simulink model "Thesis_MMC_WF_Modify"  (R2023a)
settings: Solver=VariableStepAuto  StartTime=0.0  StopTime=16  RelTol=1e-3
InitFcn:
  | % TS %
  | Ts_Control=4e-05;
  | Ts_Power=2e-05;
  | %% Main Circuit %%
  | % AC Line %
  | Vnom_Sec=333000;
  | Vnom_Pri=400000;
  | Pnom=1.0e+09;
  | Fnom=60;
  | Psc=2.0e+10;
  | P_Ld1=2/3*1e+09;
  | R_Startup=400;
  | Rxfo=0.003;
  | Lxfo=0.12;
  | P_Ld2=500e+03;
  | % MMC Parameter %
  | Larm_pu=0.15;
  | Rarm_pu=Larm_pu/100;
  | Zbase= Vnom_Sec^2/Pnom;
  | Larm=Larm_pu*(Zbase/(2*pi*Fnom));
  | Rarm=Rarm_pu*Zbase;
  | C_PM=1.758e-3;
  | w=2*pi*Fnom;
  | wc2=(2*w)^2;
  | Cfilter=1/(Larm*wc2);
  | Rfilter=1/(Cfilter*w)*30;
  | Topen_Filter=1e6;
  | K_V_dc=600000;
  | n=36;
  | Rg=100;
  | Cg=5e-08;
  | % HVDC Parameter %
  | R_cable=0.5;
  | L_cable=0.015;
  | %% Controller Parameter %%
  | % PLL %
  | Fn_filter=1000;
  | Zeta_filter=1;
  | % Active Power Regulator %
  | Kp_Preg=1/6;
  | Ki_Preg=1;
  | Limits_Preg=[0.8 1.2];
  | set_param('Thesis_MMC_WF_Modify/Controller/Active Power Regulator/Sum1','SampleTime','Ts_Control')
  | set_param('Thesis_MMC_WF_Modify/Controller/Active Power Regulator/Saturation','SampleTime','Ts_Control')
  | % Reactive Power Regulator %
  | Kp_Qreg=1/6;
  | Ki_Qreg=1;
  | Limits_Qreg=[-0.25 0.25];
  | set_param('Thesis_MMC_WF_Modify/Controller/Reactive Power Regulartor/Sum1','SampleTime','Ts_Control')
  | % Discrete Mean %
  | K1=3.2312e-30;
  | K2=-1.1369e-16;
  | Delay=0.02;
  | Vint=0;
  | Delay1=0.02004;
  | % DC Voltage Regulator %
  | Kp_VDCreg=4;
  | Ki_VDCreg=100;
  | Limits_VDCreg=[-2 2];
  | set_param('Thesis_MMC_WF_Modify/Controller/DC Voltage Regulator/Sum1','SampleTime','Ts_Control')
  | ... (+46 lines)
undefined symbols (not defined in the file): D1, Delta, Delta1, DiscIntNeverNeededParam, Lagging, Vnom_dc
libraries: spsSeriesRLCBranchLib x54, spsIGBTLib x24, spsBreakerLib x13, spsVoltageMeasurementLib x11, spsThreePhaseBreakerLib x11, spsThreePhaseVIMeasurementLib x9, spsIdealSwitchLib x8, simulink x7, spsDiscreteVariableTimeDelayLib x7, spsCurrentMeasurementLib x6, spsGroundLib x6, spsSecondOrderFilterLib x6
(part 3 of 3)

== system Thesis_MMC_WF_Modify/Controller/Current Regular/PI Regulator2 ==
  Error : Inport
  Compare To Zero : simulink/Logic and Bit Operations/Compare To Zero  relop=>  OutDataTypeStr=uint8  ZeroCross=off
  Compare To Zero1 : simulink/Logic and Bit Operations/Compare To Zero  relop=<  OutDataTypeStr=uint8  ZeroCross=off
  Constant : Constant  Value=UpperLimit
  Constant1 : Constant  Value=0
  Constant2 : Constant  Value=LowerLimit
  Discrete-Time Integrator : DiscreteIntegrator  IntegratorMethod=Integration: Trapezoidal  SampleTime=Ts_Control  LimitOutput=on  UpperSaturationLimit=UpperLimit  LowerSaturationLimit=LowerLimit  ShowStatePort=on  ICPrevOutput=DiscIntNeverNeededParam  ICPrevScaledInput=DiscIntNeverNeededParam
  Gain1 : Gain  SampleTime=Ts_Control
  Gain2 : Gain  Gain=Ki  SampleTime=Ts_Control
  Logical Operator : Logic  AllPortsSameDT=off  OutDataTypeStr=boolean
  Logical Operator1 : Logic  Operator=OR  AllPortsSameDT=off  OutDataTypeStr=boolean
  Logical Operator2 : Logic  AllPortsSameDT=off  OutDataTypeStr=boolean
  Relational Operator : RelationalOperator  Operator=<=  OutDataTypeStr=boolean  RndMeth=Simplest  InputSameDT=off
  Relational Operator1 : RelationalOperator  OutDataTypeStr=boolean  RndMeth=Simplest  InputSameDT=off
  Saturation : Saturate  UpperLimit=UpperLimit  LowerLimit=LowerLimit  SampleTime=Ts_Control
  Sum1 : Sum  SampleTime=Ts_Control
  Sum2 : Sum  SampleTime=Ts_Control
  Switch : Switch  Criteria=u2 > Threshold  SaturateOnIntegerOverflow=off  InputSameDT=off
  Zero-Order Hold : ZeroOrderHold  SampleTime=Ts_Control
  Out : Outport
  wires:
  Constant1/1 -> Switch/1
  Gain2/1 -> Switch/3
  Gain1/1 -> Zero-Order Hold/1
  Error/1 -> Compare To Zero1/1, Compare To Zero/1, Gain2/1, Gain1/1
  Switch/1 -> Discrete-Time Integrator/1
  Zero-Order Hold/1 -> Sum1/1, Sum2/2
  Discrete-Time Integrator/1 -> Sum1/2
  Sum1/1 -> Saturation/1
  Saturation/1 -> Out/1
  Sum2/1 -> Relational Operator/1, Relational Operator1/1
  Discrete-Time Integrator/State -> Sum2/1
  Constant/1 -> Relational Operator1/2
  Constant2/1 -> Relational Operator/2
  Logical Operator1/1 -> Switch/2
  Compare To Zero/1 -> Logical Operator/2
  Compare To Zero1/1 -> Logical Operator2/2
  Relational Operator1/1 -> Logical Operator/1
  Relational Operator/1 -> Logical Operator2/1
  Logical Operator2/1 -> Logical Operator1/1
  Logical Operator/1 -> Logical Operator1/2

== system Thesis_MMC_WF_Modify/Controller/PLL,Measurement and Transformation/Discrete Mean ==
  In : Inport
  Constant : Constant  Value=Delay
  Constant1 : Constant  Value=Fnom  SampleTime=Ts_Control
  Constant2 : Constant  Value=Vint
  Discrete Variable Time Delay : spsDiscreteVariableTimeDelayLib/Discrete Variable Time Delay  MaxDelay=Delay+Ts_Control  InitialValue=0  Ts=Ts_Control  DFT=on
      settings: LibrarySourceBlock=|
      | sps_lib/Control/Discrete Variable
      | Time Delay
  Discrete-Time Integrator : DiscreteIntegrator  IntegratorMethod=Integration: Trapezoidal  SampleTime=-1  ICPrevOutput=DiscIntNeverNeededParam  ICPrevScaledInput=DiscIntNeverNeededParam
  Gain1 : Gain  Gain=K1  SampleTime=Ts_Control
  Gain2 : Gain  Gain=K2  SampleTime=Ts_Control
  Product : Product
  Step : Step  Time=1/Fnom  SampleTime=Ts_Control
  Sum1 : Sum  Inputs=-+
  Sum2 : Sum  Inputs=+-
  Sum3 : Sum
  Switch : Switch  Threshold=0.5  SaturateOnIntegerOverflow=off  InputSameDT=off
  Unit Delay : UnitDelay  SampleTime=-1  HasFrameUpgradeWarning=on
  Mean : Outport
  wires:
  In/1 -> Gain2/1, Unit Delay/1, Discrete-Time Integrator/1
  Discrete-Time Integrator/1 -> Discrete Variable Time Delay/1, Sum1/2
  Constant1/1 -> Product/2
  Sum1/1 -> Product/1
  Product/1 -> Sum3/1
  Sum2/1 -> Sum3/2
  Sum3/1 -> Switch/1
  Constant2/1 -> Switch/3
  Switch/1 -> Mean/1
  Step/1 -> Switch/2
  Unit Delay/1 -> Gain1/1
  Gain1/1 -> Sum2/2
  Gain2/1 -> Sum2/1
  Discrete Variable Time Delay/1 -> Sum1/1
  Constant/1 -> Discrete Variable Time Delay/2

== system Thesis_MMC_WF_Modify/Controller/PLL,Measurement and Transformation/Discrete Mean1 ==
  In : Inport
  Constant : Constant  Value=Delay
  Constant1 : Constant  Value=Fnom  SampleTime=Ts_Control
  Constant2 : Constant  Value=Vint
  Discrete Variable Time Delay : spsDiscreteVariableTimeDelayLib/Discrete Variable Time Delay  MaxDelay=Delay+Ts_Control  InitialValue=0  Ts=Ts_Control  DFT=on
      settings: LibrarySourceBlock=|
      | sps_lib/Control/Discrete Variable
      | Time Delay
  Discrete-Time Integrator : DiscreteIntegrator  IntegratorMethod=Integration: Trapezoidal  SampleTime=-1  ICPrevOutput=DiscIntNeverNeededParam  ICPrevScaledInput=DiscIntNeverNeededParam
  Gain1 : Gain  Gain=K1  SampleTime=Ts_Control
  Gain2 : Gain  Gain=K2  SampleTime=Ts_Control
  Product : Product
  Step : Step  Time=1/Fnom  SampleTime=Ts_Control
  Sum1 : Sum  Inputs=-+
  Sum2 : Sum  Inputs=+-
  Sum3 : Sum
  Switch : Switch  Threshold=0.5  SaturateOnIntegerOverflow=off  InputSameDT=off
  Unit Delay : UnitDelay  SampleTime=-1  HasFrameUpgradeWarning=on
  Mean : Outport
  wires:
  In/1 -> Gain2/1, Unit Delay/1, Discrete-Time Integrator/1
  Discrete-Time Integrator/1 -> Discrete Variable Time Delay/1, Sum1/2
  Constant1/1 -> Product/2
  Sum1/1 -> Product/1
  Product/1 -> Sum3/1
  Sum2/1 -> Sum3/2
  Sum3/1 -> Switch/1
  Constant2/1 -> Switch/3
  Switch/1 -> Mean/1
  Step/1 -> Switch/2
  Unit Delay/1 -> Gain1/1
  Gain1/1 -> Sum2/2
  Gain2/1 -> Sum2/1
  Discrete Variable Time Delay/1 -> Sum1/1
  Constant/1 -> Discrete Variable Time Delay/2

== system Thesis_MMC_WF_Modify/Controller/PLL,Measurement1/Discrete Mean ==
  In : Inport
  Constant : Constant  Value=Delay
  Constant1 : Constant  Value=Fnom  SampleTime=Ts_Control
  Constant2 : Constant  Value=Vint
  Discrete Variable Time Delay : spsDiscreteVariableTimeDelayLib/Discrete Variable Time Delay  MaxDelay=Delay+Ts_Control  InitialValue=0  Ts=Ts_Control  DFT=on
      settings: LibrarySourceBlock=|
      | sps_lib/Control/Discrete Variable
      | Time Delay
  Discrete-Time Integrator : DiscreteIntegrator  IntegratorMethod=Integration: Trapezoidal  SampleTime=-1  ICPrevOutput=DiscIntNeverNeededParam  ICPrevScaledInput=DiscIntNeverNeededParam
  Gain1 : Gain  Gain=K1  SampleTime=Ts_Control
  Gain2 : Gain  Gain=K2  SampleTime=Ts_Control
  Product : Product
  Step : Step  Time=1/Fnom  SampleTime=Ts_Control
  Sum1 : Sum  Inputs=-+
  Sum2 : Sum  Inputs=+-
  Sum3 : Sum
  Switch : Switch  Threshold=0.5  SaturateOnIntegerOverflow=off  InputSameDT=off
  Unit Delay : UnitDelay  SampleTime=-1  HasFrameUpgradeWarning=on
  Mean : Outport
  wires:
  In/1 -> Gain2/1, Unit Delay/1, Discrete-Time Integrator/1
  Discrete-Time Integrator/1 -> Discrete Variable Time Delay/1, Sum1/2
  Constant1/1 -> Product/2
  Sum1/1 -> Product/1
  Product/1 -> Sum3/1
  Sum2/1 -> Sum3/2
  Sum3/1 -> Switch/1
  Constant2/1 -> Switch/3
  Switch/1 -> Mean/1
  Step/1 -> Switch/2
  Unit Delay/1 -> Gain1/1
  Gain1/1 -> Sum2/2
  Gain2/1 -> Sum2/1
  Discrete Variable Time Delay/1 -> Sum1/1
  Constant/1 -> Discrete Variable Time Delay/2

== system Thesis_MMC_WF_Modify/Controller/PLL,Measurement1/Discrete Mean1 ==
  In : Inport
  Constant : Constant  Value=Delay
  Constant1 : Constant  Value=Fnom  SampleTime=Ts_Control
  Constant2 : Constant  Value=Vint
  Discrete Variable Time Delay : spsDiscreteVariableTimeDelayLib/Discrete Variable Time Delay  MaxDelay=Delay+Ts_Control  InitialValue=0  Ts=Ts_Control  DFT=on
      settings: LibrarySourceBlock=|
      | sps_lib/Control/Discrete Variable
      | Time Delay
  Discrete-Time Integrator : DiscreteIntegrator  IntegratorMethod=Integration: Trapezoidal  SampleTime=-1  ICPrevOutput=DiscIntNeverNeededParam  ICPrevScaledInput=DiscIntNeverNeededParam
  Gain1 : Gain  Gain=K1  SampleTime=Ts_Control
  Gain2 : Gain  Gain=K2  SampleTime=Ts_Control
  Product : Product
  Step : Step  Time=1/Fnom  SampleTime=Ts_Control
  Sum1 : Sum  Inputs=-+
  Sum2 : Sum  Inputs=+-
  Sum3 : Sum
  Switch : Switch  Threshold=0.5  SaturateOnIntegerOverflow=off  InputSameDT=off
  Unit Delay : UnitDelay  SampleTime=-1  HasFrameUpgradeWarning=on
  Mean : Outport
  wires:
  In/1 -> Gain2/1, Unit Delay/1, Discrete-Time Integrator/1
  Discrete-Time Integrator/1 -> Discrete Variable Time Delay/1, Sum1/2
  Constant1/1 -> Product/2
  Sum1/1 -> Product/1
  Product/1 -> Sum3/1
  Sum2/1 -> Sum3/2
  Sum3/1 -> Switch/1
  Constant2/1 -> Switch/3
  Switch/1 -> Mean/1
  Step/1 -> Switch/2
  Unit Delay/1 -> Gain1/1
  Gain1/1 -> Sum2/2
  Gain2/1 -> Sum2/1
  Discrete Variable Time Delay/1 -> Sum1/1
  Constant/1 -> Discrete Variable Time Delay/2

== system Thesis_MMC_WF_Modify/Controller/PLL,Measurement2/Discrete Mean ==
  In : Inport
  Constant : Constant  Value=Delay
  Constant1 : Constant  Value=Fnom  SampleTime=Ts_Control
  Constant2 : Constant  Value=Vint
  Discrete Variable Time Delay : spsDiscreteVariableTimeDelayLib/Discrete Variable Time Delay  MaxDelay=Delay+Ts_Control  InitialValue=0  Ts=Ts_Control  DFT=on
      settings: LibrarySourceBlock=|
      | sps_lib/Control/Discrete Variable
      | Time Delay
  Discrete-Time Integrator : DiscreteIntegrator  IntegratorMethod=Integration: Trapezoidal  SampleTime=-1  ICPrevOutput=DiscIntNeverNeededParam  ICPrevScaledInput=DiscIntNeverNeededParam
  Gain1 : Gain  Gain=K1  SampleTime=Ts_Control
  Gain2 : Gain  Gain=K2  SampleTime=Ts_Control
  Product : Product
  Step : Step  Time=1/Fnom  SampleTime=Ts_Control
  Sum1 : Sum  Inputs=-+
  Sum2 : Sum  Inputs=+-
  Sum3 : Sum
  Switch : Switch  Threshold=0.5  SaturateOnIntegerOverflow=off  InputSameDT=off
  Unit Delay : UnitDelay  SampleTime=-1  HasFrameUpgradeWarning=on
  Mean : Outport
  wires:
  In/1 -> Gain2/1, Unit Delay/1, Discrete-Time Integrator/1
  Discrete-Time Integrator/1 -> Discrete Variable Time Delay/1, Sum1/2
  Constant1/1 -> Product/2
  Sum1/1 -> Product/1
  Product/1 -> Sum3/1
  Sum2/1 -> Sum3/2
  Sum3/1 -> Switch/1
  Constant2/1 -> Switch/3
  Switch/1 -> Mean/1
  Step/1 -> Switch/2
  Unit Delay/1 -> Gain1/1
  Gain1/1 -> Sum2/2
  Gain2/1 -> Sum2/1
  Discrete Variable Time Delay/1 -> Sum1/1
  Constant/1 -> Discrete Variable Time Delay/2

== system Thesis_MMC_WF_Modify/Controller/PLL,Measurement2/Discrete Mean1 ==
  In : Inport
  Constant : Constant  Value=Delay
  Constant1 : Constant  Value=Fnom  SampleTime=Ts_Control
  Constant2 : Constant  Value=Vint
  Discrete Variable Time Delay : spsDiscreteVariableTimeDelayLib/Discrete Variable Time Delay  MaxDelay=Delay+Ts_Control  InitialValue=0  Ts=Ts_Control  DFT=on
      settings: LibrarySourceBlock=|
      | sps_lib/Control/Discrete Variable
      | Time Delay
  Discrete-Time Integrator : DiscreteIntegrator  IntegratorMethod=Integration: Trapezoidal  SampleTime=-1  ICPrevOutput=DiscIntNeverNeededParam  ICPrevScaledInput=DiscIntNeverNeededParam
  Gain1 : Gain  Gain=K1  SampleTime=Ts_Control
  Gain2 : Gain  Gain=K2  SampleTime=Ts_Control
  Product : Product
  Step : Step  Time=1/Fnom  SampleTime=Ts_Control
  Sum1 : Sum  Inputs=-+
  Sum2 : Sum  Inputs=+-
  Sum3 : Sum
  Switch : Switch  Threshold=0.5  SaturateOnIntegerOverflow=off  InputSameDT=off
  Unit Delay : UnitDelay  SampleTime=-1  HasFrameUpgradeWarning=on
  Mean : Outport
  wires:
  In/1 -> Gain2/1, Unit Delay/1, Discrete-Time Integrator/1
  Discrete-Time Integrator/1 -> Discrete Variable Time Delay/1, Sum1/2
  Constant1/1 -> Product/2
  Sum1/1 -> Product/1
  Product/1 -> Sum3/1
  Sum2/1 -> Sum3/2
  Sum3/1 -> Switch/1
  Constant2/1 -> Switch/3
  Switch/1 -> Mean/1
  Step/1 -> Switch/2
  Unit Delay/1 -> Gain1/1
  Gain1/1 -> Sum2/2
  Gain2/1 -> Sum2/1
  Discrete Variable Time Delay/1 -> Sum1/1
  Constant/1 -> Discrete Variable Time Delay/2

== system Thesis_MMC_WF_Modify/Controller/PWM Generator/PWM Generator 1 ==
  Vref : Inport
  Constant1 : Constant  Value=Offse_Cr
  Constant2 : Constant  Value=Tc
  Constant3 : Constant  Value=Fc
  Data Type Conversion : DataTypeConversion  OutDataTypeStr=double  SaturateOnIntegerOverflow=off  RndMeth=Floor
  Digital Clock : DigitalClock  SampleTime=Ts_Power
  Logical Operator : Logic  Operator=NOT  AllPortsSameDT=off  OutDataTypeStr=boolean
  Lookup Table1 : Lookup  InputValues=[0 .5 1]  Table=[-1 1 -1]  LookUpMeth=Interpolation-Use End Values  SaturateOnIntegerOverflow=off
  Math Function : Math  Operator=rem
  Mux : Mux  Inputs=2
  Product : Product
  Relational Operator : RelationalOperator  OutDataTypeStr=boolean  InputSameDT=off
  Selector : Selector  InputPortWidth=2*n  IndexOptions=Index vector (dialog)  Indices=SelectPulses1  OutputSizes=1
  Sum : Sum
  P : Outport
  Cr : Outport  Port=2
  wires:
  Constant2/1 -> Math Function/2
  Math Function/1 -> Product/1
  Digital Clock/1 -> Sum/1
  Sum/1 -> Math Function/1
  Constant3/1 -> Product/2
  Product/1 -> Lookup Table1/1
  Lookup Table1/1 -> Cr/1, Relational Operator/2
  Vref/1 -> Relational Operator/1
  Relational Operator/1 -> Mux/1, Logical Operator/1
  Logical Operator/1 -> Mux/2
  Data Type Conversion/1 -> P/1
  Mux/1 -> Selector/1
  Selector/1 -> Data Type Conversion/1
  Constant1/1 -> Sum/2

== system Thesis_MMC_WF_Modify/Controller/PWM Generator/PWM Generator 2 ==
  Vref : Inport
  Constant1 : Constant  Value=Offse_Cr
  Constant2 : Constant  Value=Tc
  Constant3 : Constant  Value=Fc
  Data Type Conversion : DataTypeConversion  OutDataTypeStr=double  SaturateOnIntegerOverflow=off  RndMeth=Floor
  Digital Clock : DigitalClock  SampleTime=Ts_Power
  Logical Operator : Logic  Operator=NOT  AllPortsSameDT=off  OutDataTypeStr=boolean
  Lookup Table1 : Lookup  InputValues=[0 .5 1]  Table=[-1 1 -1]  LookUpMeth=Interpolation-Use End Values  SaturateOnIntegerOverflow=off
  Math Function : Math  Operator=rem
  Mux : Mux  Inputs=2
  Product : Product
  Relational Operator : RelationalOperator  OutDataTypeStr=boolean  InputSameDT=off
  Selector : Selector  InputPortWidth=2*n  IndexOptions=Index vector (dialog)  Indices=SelectPulses1  OutputSizes=1
  Sum : Sum
  P : Outport
  Cr : Outport  Port=2
  wires:
  Constant2/1 -> Math Function/2
  Math Function/1 -> Product/1
  Digital Clock/1 -> Sum/1
  Sum/1 -> Math Function/1
  Constant3/1 -> Product/2
  Constant1/1 -> Sum/2
  Product/1 -> Lookup Table1/1
  Lookup Table1/1 -> Cr/1, Relational Operator/2
  Vref/1 -> Relational Operator/1
  Relational Operator/1 -> Mux/1, Logical Operator/1
  Logical Operator/1 -> Mux/2
  Data Type Conversion/1 -> P/1
  Mux/1 -> Selector/1
  Selector/1 -> Data Type Conversion/1

== system Thesis_MMC_WF_Modify/Controller/PWM Generator/PWM Generator 3 ==
  Vref : Inport
  Constant1 : Constant  Value=Offse_Cr
  Constant2 : Constant  Value=Tc
  Constant3 : Constant  Value=Fc
  Data Type Conversion : DataTypeConversion  OutDataTypeStr=double  SaturateOnIntegerOverflow=off  RndMeth=Floor
  Digital Clock : DigitalClock  SampleTime=Ts_Power
  Logical Operator : Logic  Operator=NOT  AllPortsSameDT=off  OutDataTypeStr=boolean
  Lookup Table1 : Lookup  InputValues=[0 .5 1]  Table=[-1 1 -1]  LookUpMeth=Interpolation-Use End Values  SaturateOnIntegerOverflow=off
  Math Function : Math  Operator=rem
  Mux : Mux  Inputs=2
  Product : Product
  Relational Operator : RelationalOperator  OutDataTypeStr=boolean  InputSameDT=off
  Selector : Selector  InputPortWidth=2*n  IndexOptions=Index vector (dialog)  Indices=SelectPulses1  OutputSizes=1
  Sum : Sum
  P : Outport
  Cr : Outport  Port=2
  wires:
  Constant2/1 -> Math Function/2
  Math Function/1 -> Product/1
  Digital Clock/1 -> Sum/1
  Sum/1 -> Math Function/1
  Constant3/1 -> Product/2
  Constant1/1 -> Sum/2
  Product/1 -> Lookup Table1/1
  Lookup Table1/1 -> Cr/1, Relational Operator/2
  Vref/1 -> Relational Operator/1
  Relational Operator/1 -> Mux/1, Logical Operator/1
  Logical Operator/1 -> Mux/2
  Data Type Conversion/1 -> P/1
  Mux/1 -> Selector/1
  Selector/1 -> Data Type Conversion/1

== system Thesis_MMC_WF_Modify/Controller/PWM Generator/PWM Generator 4 ==
  Vref : Inport
  Constant1 : Constant  Value=Offse_Cr
  Constant2 : Constant  Value=Tc
  Constant3 : Constant  Value=Fc
  Data Type Conversion : DataTypeConversion  OutDataTypeStr=double  SaturateOnIntegerOverflow=off  RndMeth=Floor
  Digital Clock : DigitalClock  SampleTime=Ts_Power
  Logical Operator : Logic  Operator=NOT  AllPortsSameDT=off  OutDataTypeStr=boolean
  Lookup Table1 : Lookup  InputValues=[0 .5 1]  Table=[-1 1 -1]  LookUpMeth=Interpolation-Use End Values  SaturateOnIntegerOverflow=off
  Math Function : Math  Operator=rem
  Mux : Mux  Inputs=2
  Product : Product
  Relational Operator : RelationalOperator  OutDataTypeStr=boolean  InputSameDT=off
  Selector : Selector  InputPortWidth=2*n  IndexOptions=Index vector (dialog)  Indices=SelectPulses1  OutputSizes=1
  Sum : Sum
  P : Outport
  Cr : Outport  Port=2
  wires:
  Constant2/1 -> Math Function/2
  Math Function/1 -> Product/1
  Digital Clock/1 -> Sum/1
  Sum/1 -> Math Function/1
  Constant3/1 -> Product/2
  Constant1/1 -> Sum/2
  Product/1 -> Lookup Table1/1
  Lookup Table1/1 -> Cr/1, Relational Operator/2
  Vref/1 -> Relational Operator/1
  Relational Operator/1 -> Mux/1, Logical Operator/1
  Logical Operator/1 -> Mux/2
  Data Type Conversion/1 -> P/1
  Mux/1 -> Selector/1
  Selector/1 -> Data Type Conversion/1

== system Thesis_MMC_WF_Modify/Controller/PWM Generator/PWM Generator 5 ==
  Vref : Inport
  Constant1 : Constant  Value=Offse_Cr
  Constant2 : Constant  Value=Tc
  Constant3 : Constant  Value=Fc
  Data Type Conversion : DataTypeConversion  OutDataTypeStr=double  SaturateOnIntegerOverflow=off  RndMeth=Floor
  Digital Clock : DigitalClock  SampleTime=Ts_Power
  Logical Operator : Logic  Operator=NOT  AllPortsSameDT=off  OutDataTypeStr=boolean
  Lookup Table1 : Lookup  InputValues=[0 .5 1]  Table=[-1 1 -1]  LookUpMeth=Interpolation-Use End Values  SaturateOnIntegerOverflow=off
  Math Function : Math  Operator=rem
  Mux : Mux  Inputs=2
  Product : Product
  Relational Operator : RelationalOperator  OutDataTypeStr=boolean  InputSameDT=off
  Selector : Selector  InputPortWidth=2*n  IndexOptions=Index vector (dialog)  Indices=SelectPulses1  OutputSizes=1
  Sum : Sum
  P : Outport
  Cr : Outport  Port=2
  wires:
  Constant2/1 -> Math Function/2
  Math Function/1 -> Product/1
  Digital Clock/1 -> Sum/1
  Sum/1 -> Math Function/1
  Constant3/1 -> Product/2
  Constant1/1 -> Sum/2
  Product/1 -> Lookup Table1/1
  Lookup Table1/1 -> Cr/1, Relational Operator/2
  Vref/1 -> Relational Operator/1
  Relational Operator/1 -> Mux/1, Logical Operator/1
  Logical Operator/1 -> Mux/2
  Data Type Conversion/1 -> P/1
  Mux/1 -> Selector/1
  Selector/1 -> Data Type Conversion/1

== system Thesis_MMC_WF_Modify/Controller/PWM Generator/PWM Generator 6 ==
  Vref : Inport
  Constant1 : Constant  Value=Offse_Cr
  Constant2 : Constant  Value=Tc
  Constant3 : Constant  Value=Fc
  Data Type Conversion : DataTypeConversion  OutDataTypeStr=double  SaturateOnIntegerOverflow=off  RndMeth=Floor
  Digital Clock : DigitalClock  SampleTime=Ts_Power
  Logical Operator : Logic  Operator=NOT  AllPortsSameDT=off  OutDataTypeStr=boolean
  Lookup Table1 : Lookup  InputValues=[0 .5 1]  Table=[-1 1 -1]  LookUpMeth=Interpolation-Use End Values  SaturateOnIntegerOverflow=off
  Math Function : Math  Operator=rem
  Mux : Mux  Inputs=2
  Product : Product
  Relational Operator : RelationalOperator  OutDataTypeStr=boolean  InputSameDT=off
  Selector : Selector  InputPortWidth=2*n  IndexOptions=Index vector (dialog)  Indices=SelectPulses1  OutputSizes=1
  Sum : Sum
  P : Outport
  Cr : Outport  Port=2
  wires:
  Constant2/1 -> Math Function/2
  Math Function/1 -> Product/1
  Digital Clock/1 -> Sum/1
  Sum/1 -> Math Function/1
  Constant3/1 -> Product/2
  Constant1/1 -> Sum/2
  Product/1 -> Lookup Table1/1
  Lookup Table1/1 -> Cr/1, Relational Operator/2
  Vref/1 -> Relational Operator/1
  Relational Operator/1 -> Mux/1, Logical Operator/1
  Logical Operator/1 -> Mux/2
  Data Type Conversion/1 -> P/1
  Mux/1 -> Selector/1
  Selector/1 -> Data Type Conversion/1

== system Thesis_MMC_WF_Modify/Controller/Reactive Power Regulartor/Discrete Mean ==
  In : Inport
  Constant : Constant  Value=Delay
  Constant1 : Constant  Value=Fnom  SampleTime=Ts_Control
  Constant2 : Constant  Value=Vint
  Discrete Variable Time Delay : spsDiscreteVariableTimeDelayLib/Discrete Variable Time Delay  MaxDelay=Delay+Ts_Control  InitialValue=0  Ts=Ts_Control  DFT=on
      settings: LibrarySourceBlock=|
      | sps_lib/Control/Discrete Variable
      | Time Delay
  Discrete-Time Integrator : DiscreteIntegrator  IntegratorMethod=Integration: Trapezoidal  gainval=1  SampleTime=-1  ICPrevOutput=DiscIntNeverNeededParam  ICPrevScaledInput=DiscIntNeverNeededParam
  Gain1 : Gain  Gain=K1  SampleTime=Ts_Control
  Gain2 : Gain  Gain=K2  SampleTime=Ts_Control
  Product : Product
  Step : Step  Time=1/Fnom  SampleTime=Ts_Control
  Sum1 : Sum  Inputs=-+
  Sum2 : Sum  Inputs=+-
  Sum3 : Sum
  Switch : Switch  Threshold=0.5  SaturateOnIntegerOverflow=off  InputSameDT=off
  Unit Delay : UnitDelay  SampleTime=-1  HasFrameUpgradeWarning=on
  Mean : Outport
  wires:
  In/1 -> Gain2/1, Unit Delay/1, Discrete-Time Integrator/1
  Discrete-Time Integrator/1 -> Discrete Variable Time Delay/1, Sum1/2
  Constant1/1 -> Product/2
  Sum1/1 -> Product/1
  Product/1 -> Sum3/1
  Sum2/1 -> Sum3/2
  Sum3/1 -> Switch/1
  Constant2/1 -> Switch/3
  Switch/1 -> Mean/1
  Step/1 -> Switch/2
  Unit Delay/1 -> Gain1/1
  Gain1/1 -> Sum2/2
  Gain2/1 -> Sum2/1
  Discrete Variable Time Delay/1 -> Sum1/1
  Constant/1 -> Discrete Variable Time Delay/2
